simulink model "EPS_orbit_v5a"  (R2023b)
settings: Solver=FixedStepAuto  StartTime=0.0  StopTime=tsimulation  FixedStep=delta_t  RelTol=1e-3
undefined symbols (not defined in the file or in its folder): att, date, GS, juliandate, MODE, SP
libraries: dspmathops x17, vrlib x13, aerolibutil x11, sharedtransform x8, sharedutil x4, simulink_extras x1
(part 1 of 2)
settings Model: Creator=Ricardo  LastModifiedBy=lricc
settings SolverCC: AlgebraicLoopSolver=TrustRegion
settings OptimizationCC: ReuseModelBlockBuffer=off
settings DebuggingCC: UnconnectedInputMsg=warning  UnconnectedOutputMsg=warning  UnconnectedLineMsg=warning
settings ModelReferenceCC: EnableRefExpFcnMdlSchedulingChecks=on
settings RTWCC: DLArmComputeVersion=19.05

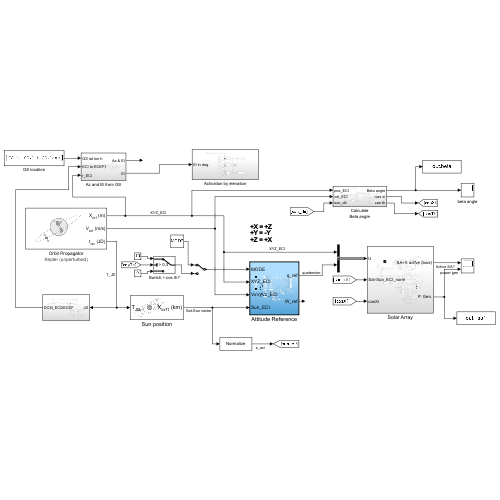
[thumbnail: Simulink's stored preview of the top-level diagram]
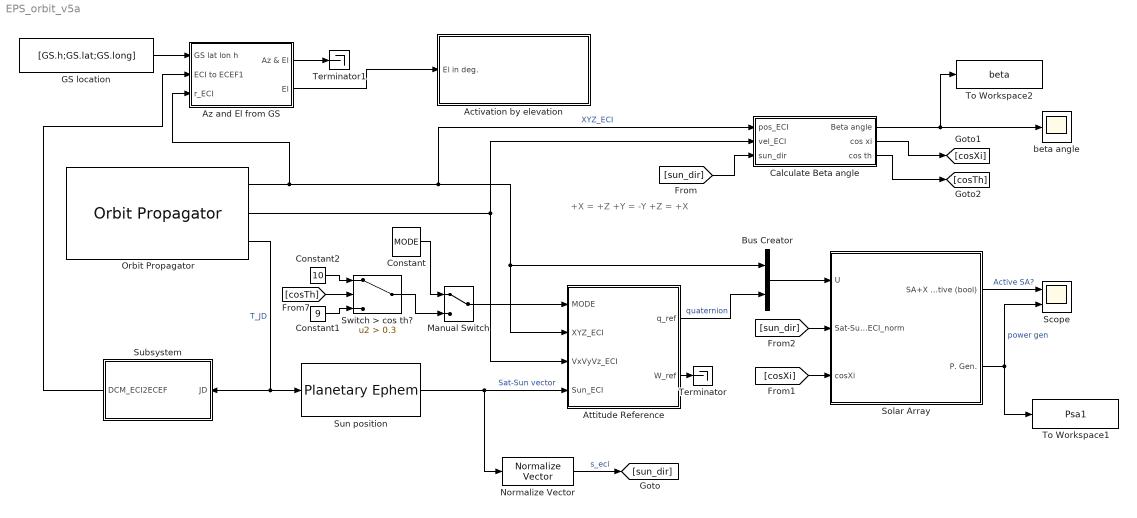
== system EPS_orbit_v5a ==
  note: +X = +Z
      | +Y = -Y
      | +Z = +X
  Activation by elevation : Subsystem
  Attitude Reference : Subsystem  TreatAsAtomicUnit=on
  Az and El from GS : Subsystem
  Bus Creator : BusCreator  Inputs=2
  Calculate Beta angle : Subsystem
  Constant : Constant  Value=MODE  OutDataTypeStr=int8
  Constant1 : Constant  Value=9
  Constant2 : Constant  Value=10
  GS location : Constant  Value=[GS.h;GS.lat;GS.long]
  Manual Switch : ManualSwitch
  Normalize Vector : vrlib/Utilities/Normalize Vector  maxzero=0
  Orbit Propagator : OrbitPropagator  startDate=juliandate(date.year, date.month, date.day, date.hour, date.minutes, date.seconds)  semiMajorAxis=orbit.a  eccentricity=orbit.e  inclination=orbit.i  raan=orbit.O  argPeriapsis=orbit.o  trueAnomaly=orbit.nu  inertialPosition=[3649700.0 3308200.0 -4676600.0]  inertialVelocity=[-2750.8 6666.4 2573.4]  fixedPosition=[-4142689.0 -2676864.7 -4669861.6]  fixedVelocity=[1452.7 -6720.7 2568.1]  customR=3396200  customMu=4.305e13  customJ2=1.0826269e-03  customOmega=4.06125949e-3
      settings: AttributesFormatString=%<propagator>
  Scope : Scope  NumInputPorts=2
  Solar Array : Subsystem
  Subsystem : Subsystem
  Sun position : PlanetaryEphem  target=Sun  outputVelocity=off
  Switch > cos th? : Switch  Criteria=u2 > Threshold  Threshold=0.3  SaturateOnIntegerOverflow=off  InputSameDT=off
  Terminator : Terminator
  Terminator1 : Terminator
  To Workspace1 : ToWorkspace  VariableName=Psa1  SaveFormat=Timeseries  SampleTime=-1
  To Workspace2 : ToWorkspace  VariableName=beta  SaveFormat=Timeseries  SampleTime=-1
  beta angle : Scope
  wires:
  Orbit Propagator/2 -> Attitude Reference/3(VxVyVz_ECI), Calculate Beta angle/2(vel_ECI)
  Orbit Propagator/1 -> Az and El from GS/3(r_ECI), Attitude Reference/2(XYZ_ECI), Bus Creator/1, Calculate Beta angle/1(pos_ECI)  "XYZ_ECI"
  Normalize Vector/1 -> [sun_dir]  "s_eci"
  Bus Creator/1 -> Solar Array/1(U)
  Sun position/1 -> Attitude Reference/4(Sun_ECI), Normalize Vector/1  "Sat-Sun vector"
  Solar Array/1(SA+X active (bool)) -> Scope/1  "Active SA?"
  Attitude Reference/1(q_ref) -> Bus Creator/2  "quaternion"
  Solar Array/2(P. Gen.) -> Scope/2, To Workspace1/1  "power gen"
  Orbit Propagator/3 -> Subsystem/1(JD), Sun position/1  "T_JD"
  Attitude Reference/2(W_ref) -> Terminator/1
  Constant/1 -> Manual Switch/1
  Calculate Beta angle/1(Beta angle) -> beta angle/1, To Workspace2/1
  [sun_dir] -> Calculate Beta angle/3(sun_dir)
  Calculate Beta angle/2(cos xi) -> [cosXi]
  [cosXi] -> Solar Array/3(cosXi)
  [sun_dir] -> Solar Array/2(Sat-Sun_ECI_norm)
  Manual Switch/1 -> Attitude Reference/1(MODE)
  Constant2/1 -> Switch > cos th?/1
  Constant1/1 -> Switch > cos th?/3
  [cosTh] -> Switch > cos th?/2
  Switch > cos th?/1 -> Manual Switch/2
  Calculate Beta angle/3(cos th) -> [cosTh]
  GS location/1 -> Az and El from GS/1(GS lat lon h)
  Subsystem/1(DCM_ECI2ECEF) -> Az and El from GS/2(ECI to ECEF1)
  Az and El from GS/1(Az & El) -> Terminator1/1
  Az and El from GS/2(El) -> Activation by elevation/1(El in deg.)

== system EPS_orbit_v5a/Activation by elevation ==
  El in deg. : Inport
  Constant1 : Constant
  Constant2 : Constant  Value=0
  Constant3 : Constant
  Constant4 : Constant  Value=0
  Constant5 : Constant
  Constant6 : Constant  Value=0
  Scope3 : Scope  NumInputPorts=3
  To Workspace1 : ToWorkspace  VariableName=el25  SaveFormat=Timeseries  SampleTime=-1
  To Workspace2 : ToWorkspace  VariableName=el00  SaveFormat=Timeseries  SampleTime=-1
  elevation>0 : Switch  Criteria=u2 > Threshold  SaturateOnIntegerOverflow=off  InputSameDT=off
  elevation>10 : Switch  Criteria=u2 > Threshold  Threshold=10  SaturateOnIntegerOverflow=off  InputSameDT=off
  elevation>25 : Switch  Criteria=u2 > Threshold  Threshold=25  SaturateOnIntegerOverflow=off  InputSameDT=off
  wires:
  Constant3/1 -> elevation>0/1
  Constant4/1 -> elevation>0/3
  elevation>0/1 -> To Workspace2/1, Scope3/1
  Constant2/1 -> elevation>10/3
  Constant1/1 -> elevation>10/1
  El in deg./1 -> elevation>25/2, elevation>10/2, elevation>0/2
  Constant6/1 -> elevation>25/3
  Constant5/1 -> elevation>25/1
  elevation>10/1 -> Scope3/2
  elevation>25/1 -> To Workspace1/1, Scope3/3

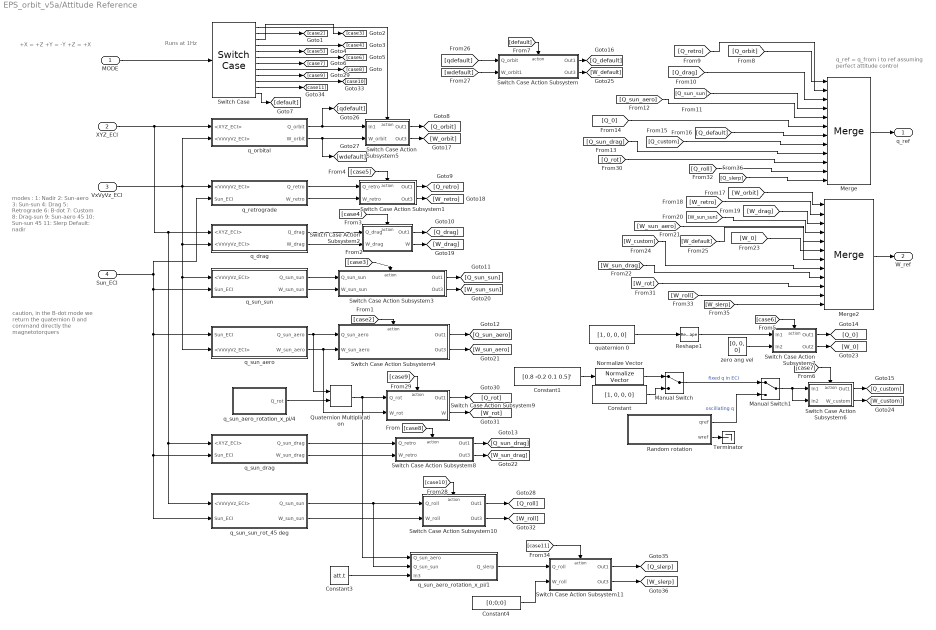
== system EPS_orbit_v5a/Attitude Reference ==
  note: caution, in the B-dot mode we return the quaternion 0 and command directly the magnetotorquers
  note: modes :
      | 1: Nadir
      | 2: Sun-aero
      | 3: Sun-sun
      | 4: Drag
      | 5: Retrograde
      | 6: B-dot
      | 7: Custom
      | 8: Drag-sun
      | 9: Sun-aero 45
      | 10: Sun-sun 45
      | 11: Slerp
      | Default: nadir
  note: q_ref  = q_from i to ref
      | assuming perfect attitude control
  note: Runs at 1Hz
  note: +X = +Z
      | +Y = -Y
      | +Z = +X
  MODE : Inport  OutMin=1  OutMax=100  OutDataTypeStr=int8
  XYZ_ECI : Inport  Port=2
  VxVyVz_ECI : Inport  Port=3
  Sun_ECI : Inport  Port=4
  Constant : Constant  Value=[1, 0, 0, 0]
  Constant1 : Constant  Value=[0.8 -0.2 0.1 0.5]'
  Constant3 : Constant  Value=att.t
  Constant4 : Constant  Value=[0;0;0]
  Manual Switch : ManualSwitch
  Manual Switch1 : ManualSwitch
  Merge : Merge  Inputs=12
  Merge2 : Merge  Inputs=12
  Normalize Vector : vrlib/Utilities/Normalize Vector  maxzero=0
  Quaternion Multiplication : aerolibutil/Quaternion Multiplication
  Random rotation : Subsystem
  Reshape1 : Reshape  OutputDimensionality=Column vector (2-D)
  Switch Case : SwitchCase  CaseConditions={1, 2, 3, 4, 5, 6, 7, 8, 9, 10, 11}
  Switch Case Action Subsystem : Subsystem  TreatAsAtomicUnit=on
  Switch Case Action Subsystem1 : Subsystem  TreatAsAtomicUnit=on
  Switch Case Action Subsystem10 : Subsystem  TreatAsAtomicUnit=on
  Switch Case Action Subsystem11 : Subsystem  TreatAsAtomicUnit=on
  Switch Case Action Subsystem2 : Subsystem  TreatAsAtomicUnit=on
  Switch Case Action Subsystem3 : Subsystem  TreatAsAtomicUnit=on
  Switch Case Action Subsystem4 : Subsystem  TreatAsAtomicUnit=on
  Switch Case Action Subsystem5 : Subsystem  TreatAsAtomicUnit=on
  Switch Case Action Subsystem6 : Subsystem  TreatAsAtomicUnit=on
  Switch Case Action Subsystem7 : Subsystem  TreatAsAtomicUnit=on
  Switch Case Action Subsystem8 : Subsystem  TreatAsAtomicUnit=on
  Switch Case Action Subsystem9 : Subsystem  TreatAsAtomicUnit=on
  Terminator : Terminator
  q_drag : Subsystem
  q_orbital : Subsystem
  q_retrograde : Subsystem
  q_sun_aero : Subsystem
  q_sun_aero_rotation_x_pi/1 : Subsystem
  q_sun_aero_rotation_x_pi/4 : Subsystem
  q_sun_drag : Subsystem
  q_sun_sun : Subsystem
  q_sun_sun_rot_45 deg : Subsystem
  quaternion 0 : Constant  Value=[1, 0, 0, 0]
  zero ang vel : Constant  Value=[0, 0, 0]
  q_ref : Outport  VectorParamsAs1DForOutWhenUnconnected=off
  W_ref : Outport  Port=2
  wires:
  quaternion 0/1 -> Reshape1/1
  Reshape1/1 -> Switch Case Action Subsystem7/1(In1)
  Constant/1 -> Manual Switch/2
  Constant1/1 -> Normalize Vector/1
  Normalize Vector/1 -> Manual Switch/1
  zero ang vel/1 -> Switch Case Action Subsystem7/2(In2)
  Manual Switch/1 -> Manual Switch1/1  "fixed q in ECI"
  Random rotation/1(qref) -> Manual Switch1/2  "oscillating q"
  Manual Switch1/1 -> Switch Case Action Subsystem6/2(In2), Switch Case Action Subsystem6/1(In1)
  [default] -> Switch Case Action Subsystem/Action
  Switch Case/7 -> [case7]
  Switch Case/4 -> [case4]
  Switch Case/5 -> [case5]
  [case3] -> Switch Case Action Subsystem3/Action
  [case5] -> Switch Case Action Subsystem1/Action
  Switch Case/3 -> [case3]
  Switch Case/2 -> [case2]
  q_drag/2(W_drag) -> Switch Case Action Subsystem2/2(W_drag)
  q_sun_drag/2(W_sun_drag) -> Switch Case Action Subsystem8/2(W_retro)
  q_sun_aero/2(W_sun_aero) -> Switch Case Action Subsystem9/2(W_rot), Switch Case Action Subsystem4/2(W_sun_aero)
  Switch Case/1 -> Switch Case Action Subsystem5/Action
  [case8] -> Switch Case Action Subsystem8/Action
  Switch Case/8 -> [case8]
  q_drag/1(Q_drag) -> Switch Case Action Subsystem2/1(Q_drag)
  Switch Case/12 -> [default]
  q_sun_sun/2(W_sun_sun) -> Switch Case Action Subsystem3/2(W_sun_sun)
  q_retrograde/2(W_retro) -> Switch Case Action Subsystem1/2(W_retro)
  q_sun_sun/1(Q_sun_sun) -> Switch Case Action Subsystem3/1(Q_sun_sun)
  q_sun_aero/1(Q_sun_aero) -> Quaternion Multiplication/1, Switch Case Action Subsystem4/1(Q_sun_aero)
  q_sun_drag/1(Q_sun_drag) -> Switch Case Action Subsystem8/1(Q_retro)
  Merge2/1 -> W_ref/1
  [case2] -> Switch Case Action Subsystem4/Action
  [case4] -> Switch Case Action Subsystem2/Action
  q_orbital/1(Q_orbit) -> [qdefault], Switch Case Action Subsystem5/1(In1)
  q_retrograde/1(Q_retro) -> Switch Case Action Subsystem1/1(Q_retro)
  q_orbital/2(W_orbit) -> [wdefault], Switch Case Action Subsystem5/2(W_orbit)
  Switch Case/6 -> [case6]
  VxVyVz_ECI/1 -> q_orbital/2(<VxVyVz_ECI>), q_retrograde/1(<VxVyVz_ECI>), q_drag/2(<VxVyVz_ECI>), q_sun_aero/2(<VxVyVz_ECI>), q_sun_sun/1(<VxVyVz_ECI>)
  Merge/1 -> q_ref/1
  MODE/1 -> Switch Case/1
  Random rotation/2(wref) -> Terminator/1
  [case6] -> Switch Case Action Subsystem7/Action
  [case7] -> Switch Case Action Subsystem6/Action
  Switch Case Action Subsystem5/1(Out1) -> [Q_orbit]
  [Q_orbit] -> Merge/1
  Switch Case Action Subsystem1/1(Out1) -> [Q_retro]
  [Q_retro] -> Merge/2
  Switch Case Action Subsystem2/1(Out1) -> [Q_drag]
  [Q_drag] -> Merge/3
  Switch Case Action Subsystem3/1(Out1) -> [Q_sun_sun]
  [Q_sun_sun] -> Merge/4
  Switch Case Action Subsystem4/1(Out1) -> [Q_sun_aero]
  [Q_sun_aero] -> Merge/5
  Switch Case Action Subsystem8/1(Out1) -> [Q_sun_drag]
  [Q_sun_drag] -> Merge/9
  Switch Case Action Subsystem7/1(Out1) -> [Q_0]
  [Q_0] -> Merge/6
  Switch Case Action Subsystem6/1(Out1) -> [Q_custom]
  [Q_custom] -> Merge/8
  Switch Case Action Subsystem/1(Out1) -> [Q_default]
  [Q_default] -> Merge/7
  Switch Case Action Subsystem5/2(Out3) -> [W_orbit]
  [W_orbit] -> Merge2/1
  Switch Case Action Subsystem1/2(Out3) -> [W_retro]
  [W_retro] -> Merge2/2
  Switch Case Action Subsystem2/2(W) -> [W_drag]
  [W_drag] -> Merge2/3
  Switch Case Action Subsystem3/2(Out3) -> [W_sun_sun]
  [W_sun_sun] -> Merge2/4
  Switch Case Action Subsystem4/2(Out3) -> [W_sun_aero]
  [W_sun_aero] -> Merge2/5
  Switch Case Action Subsystem8/2(Out3) -> [W_sun_drag]
  [W_sun_drag] -> Merge2/9
  Switch Case Action Subsystem7/2(Out2) -> [W_0]
  [W_0] -> Merge2/6
  Switch Case Action Subsystem6/2(W_custom) -> [W_custom]
  [W_custom] -> Merge2/8
  Switch Case Action Subsystem/2(Out3) -> [W_default]
  [W_default] -> Merge2/7
  [qdefault] -> Switch Case Action Subsystem/1(Q_orbit)
  [wdefault] -> Switch Case Action Subsystem/2(W_orbit1)
  q_sun_aero_rotation_x_pi/4/1(Q_rot) -> Quaternion Multiplication/2
  Quaternion Multiplication/1 -> q_sun_aero_rotation_x_pi/1/1(Q_sun_aero), Switch Case Action Subsystem9/1(Q_rot)
  Switch Case/9 -> [case9]
  [case9] -> Switch Case Action Subsystem9/Action
  Switch Case Action Subsystem9/1(Out1) -> [Q_rot]
  Switch Case Action Subsystem9/2(W) -> [W_rot]
  [Q_rot] -> Merge/10
  [W_rot] -> Merge2/10
  Sun_ECI/1 -> q_retrograde/2(Sun_ECI), q_sun_sun_rot_45 deg/2(Sun_ECI), q_sun_drag/2(Sun_ECI), q_sun_aero/1(Sun_ECI), q_sun_sun/2(Sun_ECI)
  q_sun_sun_rot_45 deg/1(Q_sun_sun) -> q_sun_aero_rotation_x_pi/1/2(Q_sun_sun), Switch Case Action Subsystem10/1(Q_roll)
  XYZ_ECI/1 -> q_sun_drag/1(<XYZ_ECI>), q_sun_sun_rot_45 deg/1(<VxVyVz_ECI>), q_drag/1(<XYZ_ECI>), q_orbital/1(<XYZ_ECI>)
  Switch Case Action Subsystem10/1(Out1) -> [Q_roll]
  [case10] -> Switch Case Action Subsystem10/Action
  q_sun_sun_rot_45 deg/2(W_sun_sun) -> Switch Case Action Subsystem10/2(W_roll)
  Switch Case Action Subsystem10/2(Out3) -> [W_roll]
  Switch Case/10 -> [case10]
  [Q_roll] -> Merge/11
  [W_roll] -> Merge2/11
  Switch Case/11 -> [case11]
  [W_slerp] -> Merge2/12
  Constant3/1 -> q_sun_aero_rotation_x_pi/1/3(In3)
  Switch Case Action Subsystem11/2(Out3) -> [W_slerp]
  [case11] -> Switch Case Action Subsystem11/Action
  Switch Case Action Subsystem11/1(Out1) -> [Q_slerp]
  q_sun_aero_rotation_x_pi/1/1(Q_slerp) -> Switch Case Action Subsystem11/1(Q_roll)
  Constant4/1 -> Switch Case Action Subsystem11/2(W_roll)
  [Q_slerp] -> Merge/12

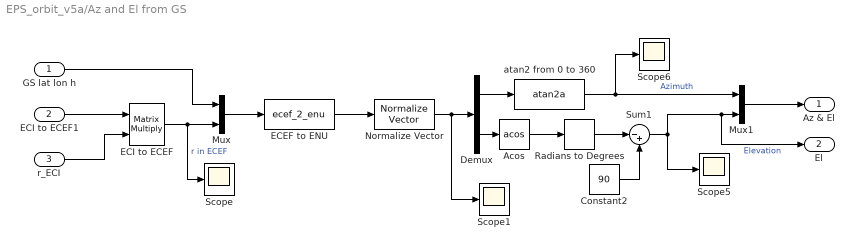
== system EPS_orbit_v5a/Az and El from GS ==
  GS lat lon h : Inport
  ECI to ECEF1 : Inport  Port=2
  r_ECI : Inport  Port=3
  Acos : Trigonometry  Operator=acos
  Constant2 : Constant  Value=90
  Demux : Demux  Outputs=[2,1]
  ECEF to ENU : MATLABFcn  MATLABFcn=ecef_2_enu  OutputDimensions=[3;1]  Output1D=off
  ECI to ECEF : Product  Multiplication=Matrix(*)
  Mux : Mux  Inputs=2
  Mux1 : Mux  Inputs=2
  Normalize Vector : vrlib/Utilities/Normalize Vector  maxzero=0
  Radians to Degrees : simulink_extras/Transformations/Radians to Degrees
  Scope{,1,5..6} (4 alike) : Scope
  Sum1 : Sum  Inputs=|-+
  atan2 from 0 to 360 : MATLABFcn  MATLABFcn=atan2a
  Az & El : Outport
  El : Outport  Port=2
  wires:
  atan2 from 0 to 360/1 -> Scope6/1, Mux1/1  "Azimuth"
  ECEF to ENU/1 -> Normalize Vector/1
  GS lat lon h/1 -> Mux/1
  Acos/1 -> Radians to Degrees/1
  ECI to ECEF1/1 -> ECI to ECEF/1
  ECI to ECEF/1 -> Scope/1, Mux/2  "r in ECEF"
  Demux/2 -> Acos/1
  Mux/1 -> ECEF to ENU/1
  Sum1/1 -> Scope5/1, El/1, Mux1/2  "Elevation"
  Normalize Vector/1 -> Scope1/1, Demux/1
  Demux/1 -> atan2 from 0 to 360/1
  Radians to Degrees/1 -> Sum1/1
  Constant2/1 -> Sum1/2
  r_ECI/1 -> ECI to ECEF/2
  Mux1/1 -> Az & El/1

== system EPS_orbit_v5a/Calculate Beta angle ==
  note: xi is calculated for the Albedo
  pos_ECI : Inport
  vel_ECI : Inport  Port=2
  sun_dir : Inport  Port=3
  Acos : Trigonometry  Operator=acos
  Constant1 : Constant  Value=90
  Cross Product : vrlib/Utilities/Cross Product
  Dot Product : DotProduct  OutDataTypeStr=Inherit: Inherit via internal rule
  Dot Product1 : DotProduct  OutDataTypeStr=Inherit: Inherit via internal rule
  Gain : Gain  Gain=180/pi
  Normalize Vector1 : vrlib/Utilities/Normalize Vector  maxzero=0
  Normalize Vector2 : vrlib/Utilities/Normalize Vector  maxzero=0
  Product : Product
  Scope : Scope  NumInputPorts=2
  Sin : Trigonometry
  Sum : Sum  Inputs=|-+
  Beta angle : Outport
  cos xi : Outport  Port=2
  cos th : Outport  Port=3
  wires:
  vel_ECI/1 -> Cross Product/2
  Dot Product/1 -> Acos/1
  Acos/1 -> Sin/1, Gain/1
  Normalize Vector1/1 -> Dot Product/2  "x"
  Gain/1 -> Sum/1
  sun_dir/1 -> Dot Product1/2, Dot Product/1
  Cross Product/1 -> Normalize Vector1/1
  Constant1/1 -> Sum/2
  pos_ECI/1 -> Normalize Vector2/1, Cross Product/1
  Sum/1 -> Beta angle/1
  Dot Product1/1 -> cos th/1, Product/2, Scope/2  "cos(theta)"
  Normalize Vector2/1 -> Dot Product1/1  "x"
  Sin/1 -> Product/1  "cos(beta)"
  Product/1 -> Scope/1, cos xi/1

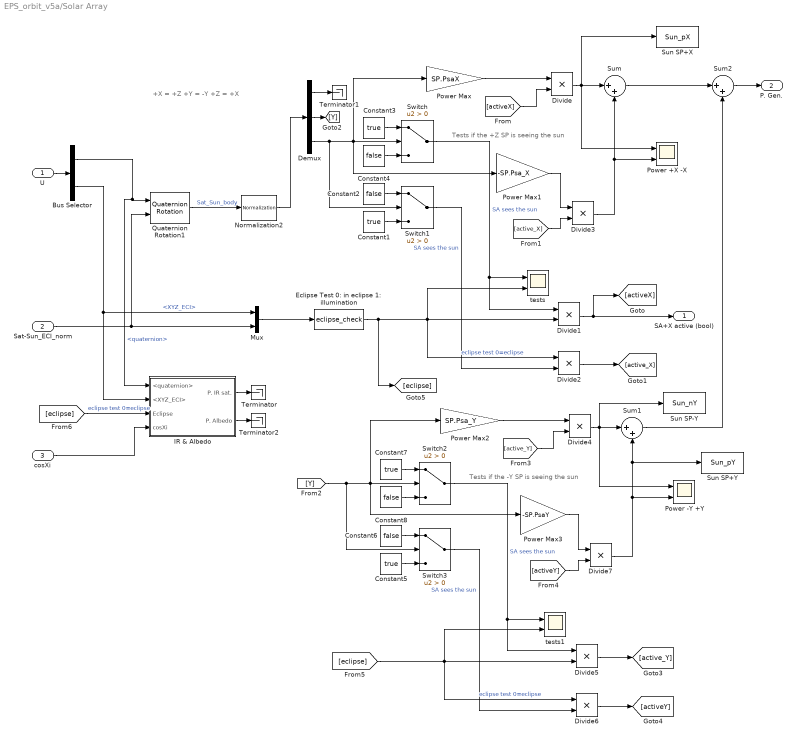
== system EPS_orbit_v5a/Solar Array ==
  note: Tests if the +Z SP is seeing the sun
  note: +X = +Z
      | +Y = -Y
      | +Z = +X
  note: Tests if the -Y SP is seeing the sun
  U : Inport
  Sat-Sun_ECI_norm : Inport  Port=2
  cosXi : Inport  Port=3
  Bus Selector : BusSelector  OutputSignals=quaternion,XYZ_ECI
  Constant{1,3,5,7} (4 alike) : Constant  Value=true
  Constant{2,4,6,8} (4 alike) : Constant  Value=false
  Demux : Demux  Outputs=3
  Divide{,1..7} (8 alike) : Product  Inputs=**
  Eclipse Test 0: in eclipse 1: illumination : MATLABFcn  MATLABFcn=eclipse_check
  IR & Albedo : Subsystem
  Mux : Mux  Inputs=2
  Normalization2 : dspmathops/Normalization  NormType=2-norm  Bias=1e-10  NormOver=Each column  Dimension=1  roundingMode=Floor  overflowMode=off  accumDataTypeStr=Inherit: Same as product output  accumLastDataTypeStr=Inherit: Same as product output  outputDataTypeStr=Inherit: Same as product output  outputMin=[]  outputMax=[]  outputLastDataTypeStr=Inherit: Same as product output
  Power +X -X : Scope  NumInputPorts=2
  Power -Y +Y : Scope  NumInputPorts=2
  Power Max : Gain  Gain=SP.PsaX
  Power Max1 : Gain  Gain=-SP.Psa_X
  Power Max2 : Gain  Gain=SP.Psa_Y
  Power Max3 : Gain  Gain=-SP.PsaY
  Quaternion Rotation1 : aerolibutil/Quaternion Rotation
  Sum : Sum  Inputs=|++
  Sum1 : Sum  Inputs=|++
  Sum2 : Sum  Inputs=|++
  Sun SP+X : ToWorkspace  VariableName=Sun_pX  SaveFormat=Timeseries  SampleTime=1
      settings: Save2DSignal=2-D array (concatenate along first dimension)
  Sun SP+Y : ToWorkspace  VariableName=Sun_pY  SaveFormat=Timeseries  SampleTime=1
      settings: Save2DSignal=2-D array (concatenate along first dimension)
  Sun SP-Y : ToWorkspace  VariableName=Sun_nY  SaveFormat=Timeseries  SampleTime=1
      settings: Save2DSignal=2-D array (concatenate along first dimension)
  Switch{,1..3} (4 alike) : Switch  Criteria=u2 > Threshold  SaturateOnIntegerOverflow=off  InputSameDT=off
  Terminator : Terminator
  Terminator1 : Terminator
  Terminator2 : Terminator
  tests : Scope  NumInputPorts=2
  tests1 : Scope  NumInputPorts=2
  SA+X active (bool) : Outport  VectorParamsAs1DForOutWhenUnconnected=off
  P. Gen. : Outport  Port=2
  wires:
  Switch/1 -> Divide1/1, tests/1  "SA sees the sun"
  U/1 -> Bus Selector/1
  Bus Selector/1 -> Quaternion Rotation1/1, IR & Albedo/1(<quaternion>)  "<quaternion>"
  Quaternion Rotation1/1 -> Normalization2/1  "Sat_Sun_body"
  Constant3/1 -> Switch/1
  Demux/2 -> [Y]
  Demux/1 -> Terminator1/1
  Bus Selector/2 -> IR & Albedo/2(<XYZ_ECI>), Mux/1  "<XYZ_ECI>"
  Divide1/1 -> [activeX], SA+X active (bool)/1
  Constant4/1 -> Switch/3
  Normalization2/1 -> Demux/1
  Divide/1 -> Sun SP+X/1, Power +X -X/1, Sum/1
  Power Max/1 -> Divide/1
  [activeX] -> Divide/2
  Sat-Sun_ECI_norm/1 -> Quaternion Rotation1/2, Mux/2
  Mux/1 -> Eclipse Test 0: in eclipse 1: illumination/1
  Eclipse Test 0: in eclipse 1: illumination/1 -> [eclipse], Divide2/1, tests/2, Divide1/2  "eclipse test 0=eclipse"
  Demux/3 -> Switch1/2, Power Max1/1, Power Max/1, Switch/2
  Constant2/1 -> Switch1/1
  Constant1/1 -> Switch1/3
  Switch1/1 -> Divide2/2  "SA sees the sun"
  Divide2/1 -> [active_X]
  [active_X] -> Divide3/2
  Power Max1/1 -> Divide3/1
  Divide3/1 -> Sum/2, Power +X -X/2
  Sum/1 -> Sum2/1
  [Y] -> Switch3/2, Power Max3/1, Power Max2/1, Switch2/2
  [eclipse] -> Divide6/1, tests1/2, Divide5/2  "eclipse test 0=eclipse"
  [active_Y] -> Divide4/2
  Constant7/1 -> Switch2/1
  Divide5/1 -> [active_Y]
  Constant8/1 -> Switch2/3
  Switch2/1 -> Divide5/1, tests1/1  "SA sees the sun"
  Sum1/1 -> Sum2/2
  Divide6/1 -> [activeY]
  Divide4/1 -> Sun SP-Y/1, Power -Y +Y/1, Sum1/1
  Switch3/1 -> Divide6/2  "SA sees the sun"
  Constant6/1 -> Switch3/1
  Power Max2/1 -> Divide4/1
  [activeY] -> Divide7/2
  Power Max3/1 -> Divide7/1
  Divide7/1 -> Power -Y +Y/2, Sun SP+Y/1, Sum1/2
  Constant5/1 -> Switch3/3
  Sum2/1 -> P. Gen./1
  [eclipse] -> IR & Albedo/3(Eclipse)  "eclipse test 0=eclipse"
  cosXi/1 -> IR & Albedo/4(cosXi)
  IR & Albedo/1(P. IR sat.) -> Terminator/1
  IR & Albedo/2(P. Albedo) -> Terminator2/1

== system EPS_orbit_v5a/Subsystem ==
  JD : Inport
  ECI_2_ECEF : MATLABFcn  MATLABFcn=eci2ecef  OutputDimensions=[3,3]  Output1D=off
  JD to UTC : MATLAB Function  TreatAsAtomicUnit=on
  Reshape : Reshape
  Scope : Scope
  Scope1 : Scope
  Signal logging : ToWorkspace  VariableName=T_UTC  SaveFormat=Timeseries  SampleTime=1
      settings: Save2DSignal=2-D array (concatenate along first dimension)
  Signal logging1 : ToWorkspace  VariableName=T_JD  SaveFormat=Timeseries  SampleTime=1
      settings: Save2DSignal=2-D array (concatenate along first dimension)
  DCM_ECI2ECEF : Outport
  wires:
  JD/1 -> Signal logging1/1, JD to UTC/1(JD)
  Reshape/1 -> Scope/1, ECI_2_ECEF/1, Signal logging/1
  JD to UTC/1(Time_UTC) -> Reshape/1
  ECI_2_ECEF/1 -> Scope1/1, DCM_ECI2ECEF/1

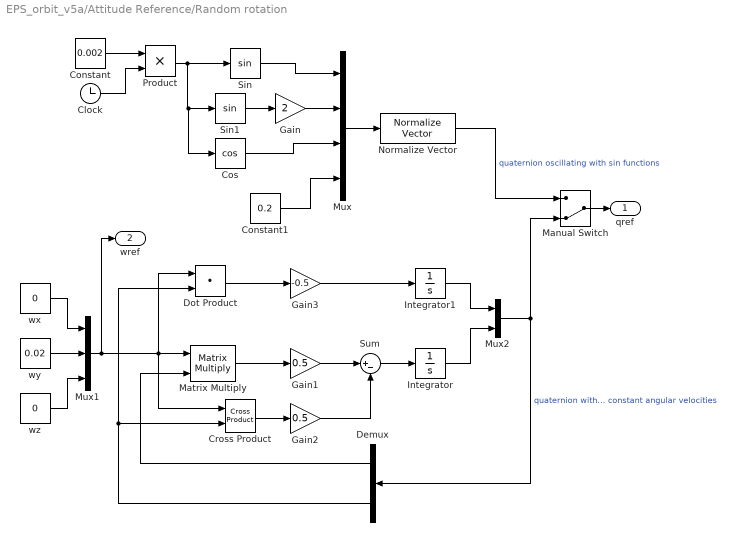
== system EPS_orbit_v5a/Attitude Reference/Random rotation ==
  Clock : Clock
      settings: Decimation=TimeStep
  Constant : Constant  Value=0.002
  Constant1 : Constant  Value=0.2
  Cos : Trigonometry  Operator=cos
  Cross Product : vrlib/Utilities/Cross Product
  Demux : Demux  Outputs=[1;3]
  Dot Product : DotProduct  OutDataTypeStr=Inherit: Inherit via internal rule
  Gain : Gain  Gain=2
  Gain1 : Gain  Gain=0.5
  Gain2 : Gain  Gain=0.5
  Gain3 : Gain  Gain=-0.5
  Integrator : Integrator  InitialCondition=[0;0;0]
  Integrator1 : Integrator  InitialCondition=1
  Manual Switch : ManualSwitch  CurrentSetting=0
  Matrix Multiply : Product  Multiplication=Matrix(*)
  Mux : Mux
  Mux1 : Mux  Inputs=3
  Mux2 : Mux  Inputs=[1;3]
  Normalize Vector : vrlib/Utilities/Normalize Vector  maxzero=0
  Product : Product
  Sin : Trigonometry
  Sin1 : Trigonometry
  Sum : Sum  Inputs=|+-
  wx : Constant  Value=0
  wy : Constant  Value=0.02
  wz : Constant  Value=0
  qref : Outport
  wref : Outport  Port=2
  wires:
  Mux/1 -> Normalize Vector/1
  Normalize Vector/1 -> Manual Switch/1  "quaternion oscillating with sin functions"
  Constant/1 -> Product/1
  Clock/1 -> Product/2
  Product/1 -> Cos/1, Sin1/1, Sin/1
  Sin/1 -> Mux/1
  Sin1/1 -> Gain/1
  Gain/1 -> Mux/2
  Cos/1 -> Mux/3
  Constant1/1 -> Mux/4
  Manual Switch/1 -> qref/1
  wx/1 -> Mux1/1
  wy/1 -> Mux1/2
  wz/1 -> Mux1/3
  Mux1/1 -> wref/1, Dot Product/1, Cross Product/1, Matrix Multiply/1
  Matrix Multiply/1 -> Gain1/1
  Gain1/1 -> Sum/1
  Sum/1 -> Integrator/1
  Integrator/1 -> Mux2/2
  Mux2/1 -> Demux/1, Manual Switch/2  "quaternion with constant angular velocities"
  Demux/1 -> Matrix Multiply/2
  Cross Product/1 -> Gain2/1
  Gain2/1 -> Sum/2
  Dot Product/1 -> Gain3/1
  Gain3/1 -> Integrator1/1
  Integrator1/1 -> Mux2/1
  Demux/2 -> Cross Product/2, Dot Product/2

== system EPS_orbit_v5a/Attitude Reference/Switch Case Action Subsystem ==
  Q_orbit : Inport
  W_orbit1 : Inport  Port=2
  Action Port : ActionPort  ActionPortLabel=default:
  Out1 : Outport  VectorParamsAs1DForOutWhenUnconnected=off
  Out3 : Outport  Port=2  VectorParamsAs1DForOutWhenUnconnected=off
  wires:
  Q_orbit/1 -> Out1/1
  W_orbit1/1 -> Out3/1

== system EPS_orbit_v5a/Attitude Reference/Switch Case Action Subsystem1 ==
  Q_retro : Inport
  W_retro : Inport  Port=2
  Action Port : ActionPort  ActionPortLabel=case [ 5 ]:
  Out1 : Outport  VectorParamsAs1DForOutWhenUnconnected=off
  Out3 : Outport  Port=2  VectorParamsAs1DForOutWhenUnconnected=off
  wires:
  Q_retro/1 -> Out1/1
  W_retro/1 -> Out3/1

== system EPS_orbit_v5a/Attitude Reference/Switch Case Action Subsystem10 ==
  note: from I to SS
  Q_roll : Inport
  W_roll : Inport  Port=2
  Action Port : ActionPort  ActionPortLabel=case [ 10 ]:
  Out1 : Outport  VectorParamsAs1DForOutWhenUnconnected=off
  Out3 : Outport  Port=2  VectorParamsAs1DForOutWhenUnconnected=off
  wires:
  Q_roll/1 -> Out1/1
  W_roll/1 -> Out3/1

== system EPS_orbit_v5a/Attitude Reference/Switch Case Action Subsystem11 ==
  note: from I to SS
  Q_roll : Inport
  W_roll : Inport  Port=2
  Action Port : ActionPort  ActionPortLabel=case [ 11 ]:
  Out1 : Outport  VectorParamsAs1DForOutWhenUnconnected=off
  Out3 : Outport  Port=2  VectorParamsAs1DForOutWhenUnconnected=off
  wires:
  Q_roll/1 -> Out1/1
  W_roll/1 -> Out3/1

== system EPS_orbit_v5a/Attitude Reference/Switch Case Action Subsystem2 ==
  note: q from I to O + rotation
  Q_drag : Inport
  W_drag : Inport  Port=2
  Action Port : ActionPort  ActionPortLabel=case [ 4 ]:
  Out1 : Outport  VectorParamsAs1DForOutWhenUnconnected=off
  W : Outport  Port=2
  wires:
  Q_drag/1 -> Out1/1
  W_drag/1 -> W/1

== system EPS_orbit_v5a/Attitude Reference/Switch Case Action Subsystem3 ==
  Q_sun_sun : Inport
  W_sun_sun : Inport  Port=2
  Action Port : ActionPort  ActionPortLabel=case [ 3 ]:
  Out1 : Outport  VectorParamsAs1DForOutWhenUnconnected=off
  Out3 : Outport  Port=2  VectorParamsAs1DForOutWhenUnconnected=off
  wires:
  Q_sun_sun/1 -> Out1/1
  W_sun_sun/1 -> Out3/1

== system EPS_orbit_v5a/Attitude Reference/Switch Case Action Subsystem4 ==
  Q_sun_aero : Inport
  W_sun_aero : Inport  Port=2
  Action Port : ActionPort  ActionPortLabel=case [ 2 ]:
  Out1 : Outport  VectorParamsAs1DForOutWhenUnconnected=off
  Out3 : Outport  Port=2  VectorParamsAs1DForOutWhenUnconnected=off
  wires:
  Q_sun_aero/1 -> Out1/1
  W_sun_aero/1 -> Out3/1

== system EPS_orbit_v5a/Attitude Reference/Switch Case Action Subsystem5 ==
  In1 : Inport
  W_orbit : Inport  Port=2
  Action Port : ActionPort  ActionPortLabel=case [ 1 ]:
  Out1 : Outport  VectorParamsAs1DForOutWhenUnconnected=off
  Out3 : Outport  Port=2  VectorParamsAs1DForOutWhenUnconnected=off
  wires:
  In1/1 -> Out1/1
  W_orbit/1 -> Out3/1

== system EPS_orbit_v5a/Attitude Reference/Switch Case Action Subsystem6 ==
  In1 : Inport
  In2 : Inport  Port=2
  Action Port : ActionPort  ActionPortLabel=case [ 7 ]:
  Derivative : Derivative
  Matrix Multiply : Product  Multiplication=Matrix(*)
  Quaternions to Direction Cosine Matrix : sharedtransform/Quaternions to  Direction Cosine Matrix  aMode=aMode
  Transpose : Math  Operator=transpose
  Transpose1 : Math  Operator=transpose
  gets vector from Skew Matrix : MATLABFcn  MATLABFcn=vec_from_skew
  Out1 : Outport  VectorParamsAs1DForOutWhenUnconnected=off
  W_custom : Outport  Port=2
  wires:
  In1/1 -> Out1/1
  In2/1 -> Quaternions to Direction Cosine Matrix/1
  Quaternions to Direction Cosine Matrix/1 -> Transpose1/1
  Matrix Multiply/1 -> gets vector from Skew Matrix/1
  Transpose/1 -> Derivative/1
  gets vector from Skew Matrix/1 -> W_custom/1
  Derivative/1 -> Matrix Multiply/1
  Transpose1/1 -> Transpose/1, Matrix Multiply/2

== system EPS_orbit_v5a/Attitude Reference/Switch Case Action Subsystem7 ==
  In1 : Inport
  In2 : Inport  Port=2
  Action Port : ActionPort  ActionPortLabel=case [ 6 ]:
  Out1 : Outport  VectorParamsAs1DForOutWhenUnconnected=off
  Out2 : Outport  Port=2  VectorParamsAs1DForOutWhenUnconnected=off
  wires:
  In1/1 -> Out1/1
  In2/1 -> Out2/1

== system EPS_orbit_v5a/Attitude Reference/Switch Case Action Subsystem8 ==
  Q_retro : Inport
  W_retro : Inport  Port=2
  Action Port : ActionPort  ActionPortLabel=case [ 8 ]:
  Out1 : Outport  VectorParamsAs1DForOutWhenUnconnected=off
  Out3 : Outport  Port=2  VectorParamsAs1DForOutWhenUnconnected=off
  wires:
  Q_retro/1 -> Out1/1
  W_retro/1 -> Out3/1

== system EPS_orbit_v5a/Attitude Reference/Switch Case Action Subsystem9 ==
  note: q from I to O + rotation
  Q_rot : Inport
  W_rot : Inport  Port=2
  Action Port : ActionPort  ActionPortLabel=case [ 9 ]:
  Out1 : Outport  VectorParamsAs1DForOutWhenUnconnected=off
  W : Outport  Port=2
  wires:
  Q_rot/1 -> Out1/1
  W_rot/1 -> W/1

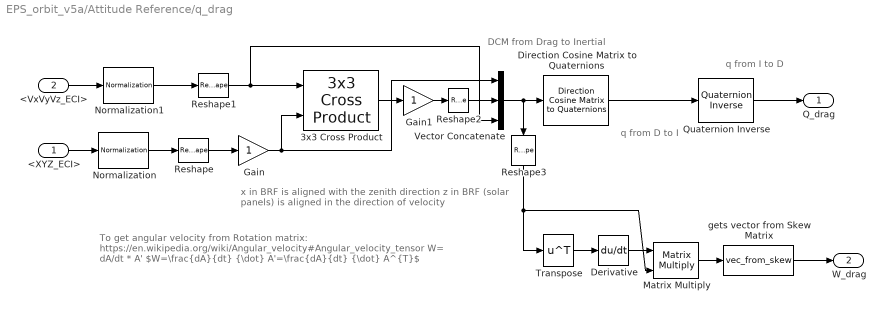
== system EPS_orbit_v5a/Attitude Reference/q_drag ==
  note: x in BRF is aligned with the zenith direction
      | z in BRF (solar panels) is aligned in the direction of velocity
  note: DCM from Drag to Inertial
  note: q from D to I
  note: q from I to D
  note: To get angular velocity from Rotation matrix:
      | https://en.wikipedia.org/wiki/Angular_velocity#Angular_velocity_tensor
      | W= dA/dt * A'
      | $W=\frac{dA}{dt} {\dot} A'=\frac{dA}{dt} {\dot} A^{T}$
  <XYZ_ECI> : Inport
  <VxVyVz_ECI> : Inport  Port=2
  3x3 Cross Product : sharedutil/3x3 Cross Product  aMode=aMode
  Derivative : Derivative
  Direction Cosine Matrix to Quaternions : sharedtransform/Direction Cosine Matrix  to Quaternions  aMode=0  action=None  tolerance=eps(2)
  Gain : Gain
  Gain1 : Gain
  Matrix Multiply : Product  Multiplication=Matrix(*)
  Normalization : dspmathops/Normalization  NormType=2-norm  Bias=1e-10  NormOver=Each column  Dimension=1  roundingMode=Floor  overflowMode=off  accumDataTypeStr=Inherit: Same as product output  accumLastDataTypeStr=Inherit: Same as product output  outputDataTypeStr=Inherit: Same as product output  outputMin=[]  outputMax=[]  outputLastDataTypeStr=Inherit: Same as product output
  Normalization1 : dspmathops/Normalization  NormType=2-norm  Bias=1e-10  NormOver=Each column  Dimension=1  roundingMode=Floor  overflowMode=off  accumDataTypeStr=Inherit: Same as product output  accumLastDataTypeStr=Inherit: Same as product output  outputDataTypeStr=Inherit: Same as product output  outputMin=[]  outputMax=[]  outputLastDataTypeStr=Inherit: Same as product output
  Quaternion Inverse : aerolibutil/Quaternion Inverse
  Reshape : Reshape  OutputDimensionality=Column vector (2-D)
  Reshape1 : Reshape  OutputDimensionality=Column vector (2-D)
  Reshape2 : Reshape  OutputDimensionality=Column vector (2-D)
  Reshape3 : Reshape  OutputDimensionality=Customize  OutputDimensions=[3,3]
  Transpose : Math  Operator=transpose
  Vector Concatenate : Concatenate  NumInputs=3  Mode=Multidimensional array  ConcatenateDimension=2
  gets vector from Skew Matrix : MATLABFcn  MATLABFcn=vec_from_skew
  Q_drag : Outport  VectorParamsAs1DForOutWhenUnconnected=off
  W_drag : Outport  Port=2
  wires:
  Normalization/1 -> Reshape/1
  Normalization1/1 -> Reshape1/1
  <VxVyVz_ECI>/1 -> Normalization1/1
  Reshape1/1 -> Vector Concatenate/3, 3x3 Cross Product/1
  <XYZ_ECI>/1 -> Normalization/1
  Reshape/1 -> Gain/1
  Gain/1 -> Vector Concatenate/1, 3x3 Cross Product/2
  Direction Cosine Matrix to Quaternions/1 -> Quaternion Inverse/1
  3x3 Cross Product/1 -> Gain1/1
  Gain1/1 -> Reshape2/1
  Quaternion Inverse/1 -> Q_drag/1
  Vector Concatenate/1 -> Reshape3/1, Direction Cosine Matrix to Quaternions/1
  gets vector from Skew Matrix/1 -> W_drag/1
  Matrix Multiply/1 -> gets vector from Skew Matrix/1
  Transpose/1 -> Derivative/1
  Derivative/1 -> Matrix Multiply/1
  Reshape2/1 -> Vector Concatenate/2
  Reshape3/1 -> Matrix Multiply/2, Transpose/1

== system EPS_orbit_v5a/Attitude Reference/q_orbital ==
  note: DCM from Orbital to Inertial
  note: q from O to I
  note: q from I to O
  note: To get angular velocity from Rotation matrix:
      | https://en.wikipedia.org/wiki/Angular_velocity#Angular_velocity_tensor
      | W= dA/dt * A'
      | $W=\frac{dA}{dt} {\dot} A'=\frac{dA}{dt} {\dot} A^{T}$
  <XYZ_ECI> : Inport
  <VxVyVz_ECI> : Inport  Port=2
  3x3 Cross Product : sharedutil/3x3 Cross Product  aMode=aMode
  Derivative : Derivative
  Direction Cosine Matrix to Quaternions : sharedtransform/Direction Cosine Matrix  to Quaternions  aMode=0  action=None  tolerance=eps(2)
  Gain : Gain
  Gain1 : Gain  Gain=-1
  Matrix Multiply : Product  Multiplication=Matrix(*)
  Normalization : dspmathops/Normalization  NormType=2-norm  Bias=1e-10  NormOver=Each column  Dimension=1  roundingMode=Floor  overflowMode=off  accumDataTypeStr=Inherit: Same as product output  accumLastDataTypeStr=Inherit: Same as product output  outputDataTypeStr=Inherit: Same as product output  outputMin=[]  outputMax=[]  outputLastDataTypeStr=Inherit: Same as product output
  Normalization1 : dspmathops/Normalization  NormType=2-norm  Bias=1e-10  NormOver=Each column  Dimension=1  roundingMode=Floor  overflowMode=off  accumDataTypeStr=Inherit: Same as product output  accumLastDataTypeStr=Inherit: Same as product output  outputDataTypeStr=Inherit: Same as product output  outputMin=[]  outputMax=[]  outputLastDataTypeStr=Inherit: Same as product output
  Quaternion Inverse : aerolibutil/Quaternion Inverse
  Reshape : Reshape  OutputDimensionality=Column vector (2-D)
  Reshape1 : Reshape  OutputDimensionality=Column vector (2-D)
  Reshape2 : Reshape  OutputDimensionality=Column vector (2-D)
  Reshape3 : Reshape  OutputDimensionality=Customize  OutputDimensions=[3,3]
  Transpose : Math  Operator=transpose
  Vector Concatenate : Concatenate  NumInputs=3  Mode=Multidimensional array  ConcatenateDimension=2
  gets vector from Skew Matrix : MATLABFcn  MATLABFcn=vec_from_skew
  Q_orbit : Outport  VectorParamsAs1DForOutWhenUnconnected=off
  W_orbit : Outport  Port=2
  wires:
  Normalization/1 -> Reshape/1
  Normalization1/1 -> Reshape1/1
  <VxVyVz_ECI>/1 -> Normalization1/1
  Reshape1/1 -> 3x3 Cross Product/1, Vector Concatenate/1
  <XYZ_ECI>/1 -> Normalization/1
  Reshape/1 -> Gain/1
  Gain/1 -> 3x3 Cross Product/2, Vector Concatenate/3
  Direction Cosine Matrix to Quaternions/1 -> Quaternion Inverse/1
  3x3 Cross Product/1 -> Gain1/1
  Gain1/1 -> Reshape2/1
  Quaternion Inverse/1 -> Q_orbit/1
  Vector Concatenate/1 -> Reshape3/1, Direction Cosine Matrix to Quaternions/1
  gets vector from Skew Matrix/1 -> W_orbit/1
  Matrix Multiply/1 -> gets vector from Skew Matrix/1
  Transpose/1 -> Derivative/1
  Derivative/1 -> Matrix Multiply/1
  Reshape2/1 -> Vector Concatenate/2
  Reshape3/1 -> Matrix Multiply/2, Transpose/1

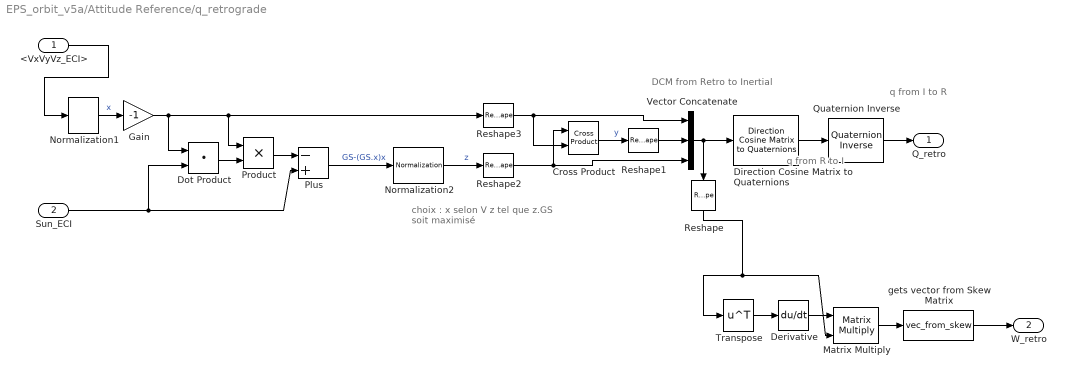
== system EPS_orbit_v5a/Attitude Reference/q_retrograde ==
  note: q from I to R
  note: q from R to I
  note: DCM from Retro to Inertial
  note: choix :
      | x selon V
      | z tel que z.GS soit maximisé
  <VxVyVz_ECI> : Inport
  Sun_ECI : Inport  Port=2
  Cross Product : vrlib/Utilities/Cross Product
  Derivative : Derivative
  Direction Cosine Matrix to Quaternions : sharedtransform/Direction Cosine Matrix  to Quaternions  aMode=0  action=None  tolerance=eps(2)
  Dot Product : DotProduct  OutDataTypeStr=Inherit: Inherit via internal rule
  Gain : Gain  Gain=-1
  Matrix Multiply : Product  Multiplication=Matrix(*)
  Normalization1 : dspmathops/Normalization  NormType=2-norm  Bias=1e-10  NormOver=Each column  Dimension=1  roundingMode=Floor  overflowMode=off  accumDataTypeStr=Inherit: Same as product output  accumLastDataTypeStr=Inherit: Same as product output  outputDataTypeStr=Inherit: Same as product output  outputMin=[]  outputMax=[]  outputLastDataTypeStr=Inherit: Same as product output
  Normalization2 : dspmathops/Normalization  NormType=2-norm  Bias=1e-10  NormOver=Each column  Dimension=1  roundingMode=Floor  overflowMode=off  accumDataTypeStr=Inherit: Same as product output  accumLastDataTypeStr=Inherit: Same as product output  outputDataTypeStr=Inherit: Same as product output  outputMin=[]  outputMax=[]  outputLastDataTypeStr=Inherit: Same as product output
  Plus : Sum  Inputs=-+
  Product : Product
  Quaternion Inverse : aerolibutil/Quaternion Inverse
  Reshape : Reshape  OutputDimensionality=Customize  OutputDimensions=[3,3]
  Reshape1 : Reshape  OutputDimensionality=Column vector (2-D)
  Reshape2 : Reshape  OutputDimensionality=Column vector (2-D)
  Reshape3 : Reshape  OutputDimensionality=Column vector (2-D)
  Transpose : Math  Operator=transpose
  Vector Concatenate : Concatenate  NumInputs=3  Mode=Multidimensional array  ConcatenateDimension=2
  gets vector from Skew Matrix : MATLABFcn  MATLABFcn=vec_from_skew
  Q_retro : Outport  VectorParamsAs1DForOutWhenUnconnected=off
  W_retro : Outport  Port=2
  wires:
  Quaternion Inverse/1 -> Q_retro/1
  Reshape2/1 -> Vector Concatenate/3, Cross Product/1
  Reshape3/1 -> Vector Concatenate/1, Cross Product/2
  Product/1 -> Plus/1
  Dot Product/1 -> Product/2
  Cross Product/1 -> Reshape1/1  "y"
  Normalization2/1 -> Reshape2/1  "z"
  Plus/1 -> Normalization2/1  "GS-(GS.x)x"
  Sun_ECI/1 -> Dot Product/2, Plus/2
  Direction Cosine Matrix to Quaternions/1 -> Quaternion Inverse/1
  Normalization1/1 -> Gain/1  "x"
  <VxVyVz_ECI>/1 -> Normalization1/1
  Reshape1/1 -> Vector Concatenate/2
  Gain/1 -> Dot Product/1, Product/1, Reshape3/1
  Vector Concatenate/1 -> Direction Cosine Matrix to Quaternions/1, Reshape/1
  gets vector from Skew Matrix/1 -> W_retro/1
  Matrix Multiply/1 -> gets vector from Skew Matrix/1
  Derivative/1 -> Matrix Multiply/1
  Transpose/1 -> Derivative/1
  Reshape/1 -> Transpose/1, Matrix Multiply/2

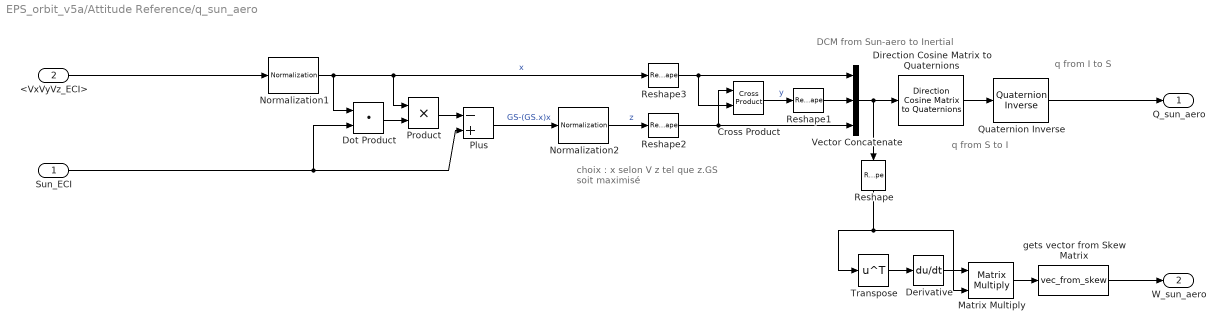
== system EPS_orbit_v5a/Attitude Reference/q_sun_aero ==
  note: q from I to S
  note: q from S to I
  note: DCM from Sun-aero to Inertial
  note: choix :
      | x selon V
      | z tel que z.GS soit maximisé
  Sun_ECI : Inport
  <VxVyVz_ECI> : Inport  Port=2
  Cross Product : vrlib/Utilities/Cross Product
  Derivative : Derivative
  Direction Cosine Matrix to Quaternions : sharedtransform/Direction Cosine Matrix  to Quaternions  aMode=0  action=None  tolerance=eps(2)
  Dot Product : DotProduct  OutDataTypeStr=Inherit: Inherit via internal rule
  Matrix Multiply : Product  Multiplication=Matrix(*)
  Normalization1 : dspmathops/Normalization  NormType=2-norm  Bias=1e-10  NormOver=Each column  Dimension=1  roundingMode=Floor  overflowMode=off  accumDataTypeStr=Inherit: Same as product output  accumLastDataTypeStr=Inherit: Same as product output  outputDataTypeStr=Inherit: Same as product output  outputMin=[]  outputMax=[]  outputLastDataTypeStr=Inherit: Same as product output
  Normalization2 : dspmathops/Normalization  NormType=2-norm  Bias=1e-10  NormOver=Each column  Dimension=1  roundingMode=Floor  overflowMode=off  accumDataTypeStr=Inherit: Same as product output  accumLastDataTypeStr=Inherit: Same as product output  outputDataTypeStr=Inherit: Same as product output  outputMin=[]  outputMax=[]  outputLastDataTypeStr=Inherit: Same as product output
  Plus : Sum  Inputs=-+
  Product : Product
  Quaternion Inverse : aerolibutil/Quaternion Inverse
  Reshape : Reshape  OutputDimensionality=Customize  OutputDimensions=[3,3]
  Reshape1 : Reshape  OutputDimensionality=Column vector (2-D)
  Reshape2 : Reshape  OutputDimensionality=Column vector (2-D)
  Reshape3 : Reshape  OutputDimensionality=Column vector (2-D)
  Transpose : Math  Operator=transpose
  Vector Concatenate : Concatenate  NumInputs=3  Mode=Multidimensional array  ConcatenateDimension=2
  gets vector from Skew Matrix : MATLABFcn  MATLABFcn=vec_from_skew
  Q_sun_aero : Outport  VectorParamsAs1DForOutWhenUnconnected=off
  W_sun_aero : Outport  Port=2
  wires:
  Reshape2/1 -> Vector Concatenate/3, Cross Product/1
  Reshape3/1 -> Vector Concatenate/1, Cross Product/2
  Product/1 -> Plus/1
  Dot Product/1 -> Product/2
  Cross Product/1 -> Reshape1/1  "y"
  Normalization2/1 -> Reshape2/1  "z"
  Plus/1 -> Normalization2/1  "GS-(GS.x)x"
  Sun_ECI/1 -> Dot Product/2, Plus/2
  Direction Cosine Matrix to Quaternions/1 -> Quaternion Inverse/1
  Normalization1/1 -> Dot Product/1, Product/1, Reshape3/1  "x"
  <VxVyVz_ECI>/1 -> Normalization1/1
  Reshape1/1 -> Vector Concatenate/2
  Transpose/1 -> Derivative/1
  Matrix Multiply/1 -> gets vector from Skew Matrix/1
  Derivative/1 -> Matrix Multiply/1
  Vector Concatenate/1 -> Direction Cosine Matrix to Quaternions/1, Reshape/1
  gets vector from Skew Matrix/1 -> W_sun_aero/1
  Reshape/1 -> Transpose/1, Matrix Multiply/2
  Quaternion Inverse/1 -> Q_sun_aero/1

== system EPS_orbit_v5a/Attitude Reference/q_sun_aero_rotation_x_pi//1 ==
  Q_sun_aero : Inport
  Q_sun_sun : Inport  Port=2
  In3 : Inport  Port=3
  Quaternion Interpolation : QuatInterp
  Quaternion Normalize : sharedutil/Quaternion Normalize  aMode=aMode
  Quaternion Normalize1 : sharedutil/Quaternion Normalize  aMode=aMode
  Q_slerp : Outport  VectorParamsAs1DForOutWhenUnconnected=off
  wires:
  Quaternion Interpolation/1 -> Q_slerp/1
  Q_sun_sun/1 -> Quaternion Normalize1/1
  Q_sun_aero/1 -> Quaternion Normalize/1
  In3/1 -> Quaternion Interpolation/3
  Quaternion Normalize/1 -> Quaternion Interpolation/1
  Quaternion Normalize1/1 -> Quaternion Interpolation/2

== system EPS_orbit_v5a/Attitude Reference/q_sun_aero_rotation_x_pi//4 ==
  note: switch top position: no 'attitude error'
  note: this is a rotation of 45 degrees around X axis
      | to maximize the power generation, exposing faces
      | X and Y to the sun
  note: this is a rotation of 15 degrees around one axis
      | to simulate off-pointing for the power generation,
  Constant : Constant  Value=[1;0;0]
  Constant1 : Constant  Value=att.offset_axis
  Manual Switch : ManualSwitch  CurrentSetting=0
  Product : Product
  Product1 : Product
  Quaternion Multiplication : aerolibutil/Quaternion Multiplication
  Reshape1 : Reshape  OutputDimensionality=Column vector (2-D)
  Reshape2 : Reshape  OutputDimensionality=Column vector (2-D)
  Vector Concatenate1 : Concatenate  Mode=Multidimensional array
  Vector Concatenate2 : Concatenate  Mode=Multidimensional array
  cos 15 : Constant  Value=[cos(-att.offset_angle/2)]
  cos pi/2 : Constant  Value=[cos(-att.angle_roll/2)]
  sin 15 : Constant  Value=sin(-att.offset_angle/2)
  sin pi/4 : Constant  Value=sin(-att.angle_roll/2)
  Q_rot : Outport  VectorParamsAs1DForOutWhenUnconnected=off
  wires:
  cos pi/2/1 -> Vector Concatenate1/1
  Manual Switch/1 -> Q_rot/1
  sin pi/4/1 -> Product/2
  Product/1 -> Reshape1/1
  Reshape1/1 -> Vector Concatenate1/2
  Constant/1 -> Product/1  "x"
  Vector Concatenate1/1 -> Quaternion Multiplication/1, Manual Switch/1
  Product1/1 -> Reshape2/1
  cos 15/1 -> Vector Concatenate2/1
  Reshape2/1 -> Vector Concatenate2/2
  Constant1/1 -> Product1/1  "y"
  sin 15/1 -> Product1/2
  Vector Concatenate2/1 -> Quaternion Multiplication/2
  Quaternion Multiplication/1 -> Manual Switch/2

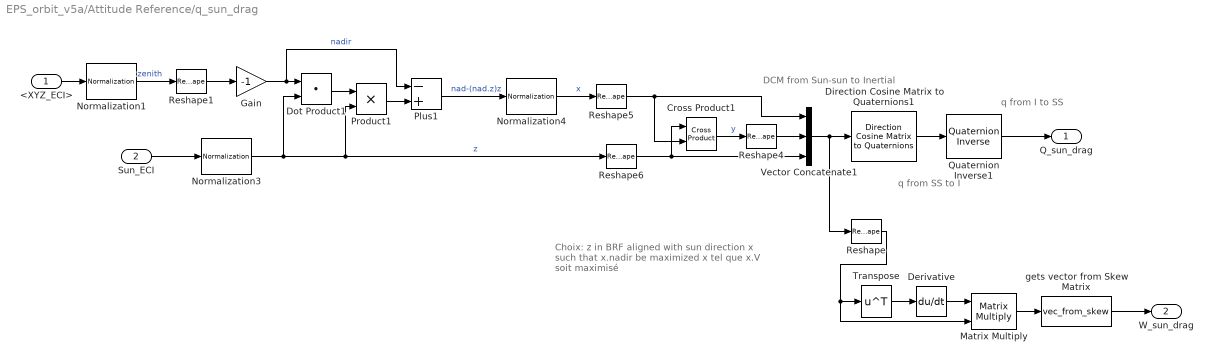
== system EPS_orbit_v5a/Attitude Reference/q_sun_drag ==
  note: Choix:
      | z in BRF aligned with sun direction
      | x such that x.nadir be maximized
      | x tel que x.V soit maximisé
  note: DCM from Sun-sun to Inertial
  note: q from I to SS
  note: q from SS to I
  <XYZ_ECI> : Inport
  Sun_ECI : Inport  Port=2
  Cross Product1 : vrlib/Utilities/Cross Product
  Derivative : Derivative
  Direction Cosine Matrix to Quaternions1 : sharedtransform/Direction Cosine Matrix  to Quaternions  aMode=0  action=None  tolerance=eps(2)
  Dot Product1 : DotProduct  OutDataTypeStr=Inherit: Inherit via internal rule
  Gain : Gain  Gain=-1
  Matrix Multiply : Product  Multiplication=Matrix(*)
  Normalization1 : dspmathops/Normalization  NormType=2-norm  Bias=1e-10  NormOver=Each column  Dimension=1  roundingMode=Floor  overflowMode=off  accumDataTypeStr=Inherit: Same as product output  accumLastDataTypeStr=Inherit: Same as product output  outputDataTypeStr=Inherit: Same as product output  outputMin=[]  outputMax=[]  outputLastDataTypeStr=Inherit: Same as product output
  Normalization3 : dspmathops/Normalization  NormType=2-norm  Bias=1e-10  NormOver=Each column  Dimension=1  roundingMode=Floor  overflowMode=off  accumDataTypeStr=Inherit: Same as product output  accumLastDataTypeStr=Inherit: Same as product output  outputDataTypeStr=Inherit: Same as product output  outputMin=[]  outputMax=[]  outputLastDataTypeStr=Inherit: Same as product output
  Normalization4 : dspmathops/Normalization  NormType=2-norm  Bias=1e-10  NormOver=Each column  Dimension=1  roundingMode=Floor  overflowMode=off  accumDataTypeStr=Inherit: Same as product output  accumLastDataTypeStr=Inherit: Same as product output  outputDataTypeStr=Inherit: Same as product output  outputMin=[]  outputMax=[]  outputLastDataTypeStr=Inherit: Same as product output
  Plus1 : Sum  Inputs=-+
  Product1 : Product
  Quaternion Inverse1 : aerolibutil/Quaternion Inverse
  Reshape : Reshape  OutputDimensionality=Customize  OutputDimensions=[3,3]
  Reshape{1,4..6} (4 alike) : Reshape  OutputDimensionality=Column vector (2-D)
  Transpose : Math  Operator=transpose
  Vector Concatenate1 : Concatenate  NumInputs=3  Mode=Multidimensional array  ConcatenateDimension=2
  gets vector from Skew Matrix : MATLABFcn  MATLABFcn=vec_from_skew
  Q_sun_drag : Outport  VectorParamsAs1DForOutWhenUnconnected=off
  W_sun_drag : Outport  Port=2
  wires:
  Direction Cosine Matrix to Quaternions1/1 -> Quaternion Inverse1/1
  Reshape4/1 -> Vector Concatenate1/2
  Dot Product1/1 -> Product1/1
  Sun_ECI/1 -> Normalization3/1
  Quaternion Inverse1/1 -> Q_sun_drag/1
  Reshape1/1 -> Gain/1
  Plus1/1 -> Normalization4/1  "nad-(nad.z)z"
  Reshape6/1 -> Cross Product1/1, Vector Concatenate1/3
  Normalization3/1 -> Dot Product1/2, Product1/2, Reshape6/1  "z"
  Reshape5/1 -> Cross Product1/2, Vector Concatenate1/1
  Cross Product1/1 -> Reshape4/1  "y"
  Normalization4/1 -> Reshape5/1  "x"
  Product1/1 -> Plus1/2
  Reshape/1 -> Matrix Multiply/2, Transpose/1
  Derivative/1 -> Matrix Multiply/1
  Transpose/1 -> Derivative/1
  Matrix Multiply/1 -> gets vector from Skew Matrix/1
  gets vector from Skew Matrix/1 -> W_sun_drag/1
  Vector Concatenate1/1 -> Direction Cosine Matrix to Quaternions1/1, Reshape/1
  <XYZ_ECI>/1 -> Normalization1/1
  Normalization1/1 -> Reshape1/1  "zenith"
  Gain/1 -> Dot Product1/1, Plus1/1  "nadir"

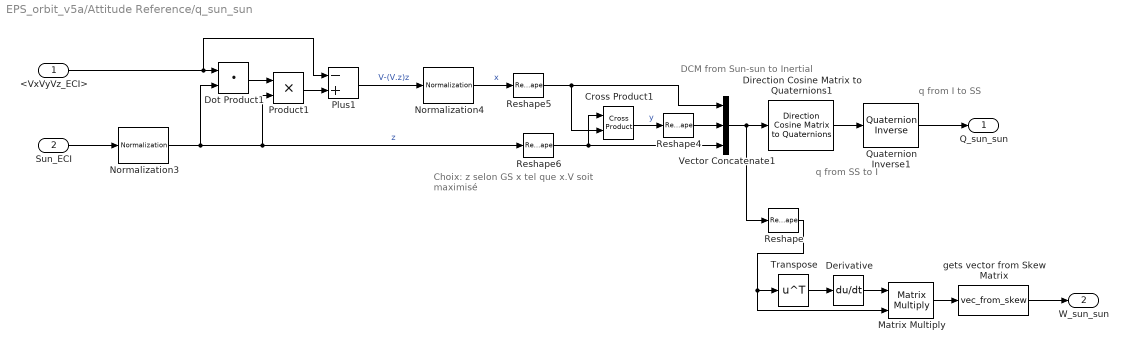
== system EPS_orbit_v5a/Attitude Reference/q_sun_sun ==
  note: Choix:
      | z selon GS
      | x tel que x.V soit maximisé
  note: DCM from Sun-sun to Inertial
  note: q from I to SS
  note: q from SS to I
  <VxVyVz_ECI> : Inport
  Sun_ECI : Inport  Port=2
  Cross Product1 : vrlib/Utilities/Cross Product
  Derivative : Derivative
  Direction Cosine Matrix to Quaternions1 : sharedtransform/Direction Cosine Matrix  to Quaternions  aMode=0  action=None  tolerance=eps(2)
  Dot Product1 : DotProduct  OutDataTypeStr=Inherit: Inherit via internal rule
  Matrix Multiply : Product  Multiplication=Matrix(*)
  Normalization3 : dspmathops/Normalization  NormType=2-norm  Bias=1e-10  NormOver=Each column  Dimension=1  roundingMode=Floor  overflowMode=off  accumDataTypeStr=Inherit: Same as product output  accumLastDataTypeStr=Inherit: Same as product output  outputDataTypeStr=Inherit: Same as product output  outputMin=[]  outputMax=[]  outputLastDataTypeStr=Inherit: Same as product output
  Normalization4 : dspmathops/Normalization  NormType=2-norm  Bias=1e-10  NormOver=Each column  Dimension=1  roundingMode=Floor  overflowMode=off  accumDataTypeStr=Inherit: Same as product output  accumLastDataTypeStr=Inherit: Same as product output  outputDataTypeStr=Inherit: Same as product output  outputMin=[]  outputMax=[]  outputLastDataTypeStr=Inherit: Same as product output
  Plus1 : Sum  Inputs=-+
  Product1 : Product
  Quaternion Inverse1 : aerolibutil/Quaternion Inverse
  Reshape : Reshape  OutputDimensionality=Customize  OutputDimensions=[3,3]
  Reshape4 : Reshape  OutputDimensionality=Column vector (2-D)
  Reshape5 : Reshape  OutputDimensionality=Column vector (2-D)
  Reshape6 : Reshape  OutputDimensionality=Column vector (2-D)
  Transpose : Math  Operator=transpose
  Vector Concatenate1 : Concatenate  NumInputs=3  Mode=Multidimensional array  ConcatenateDimension=2
  gets vector from Skew Matrix : MATLABFcn  MATLABFcn=vec_from_skew
  Q_sun_sun : Outport  VectorParamsAs1DForOutWhenUnconnected=off
  W_sun_sun : Outport  Port=2
  wires:
  Direction Cosine Matrix to Quaternions1/1 -> Quaternion Inverse1/1
  Reshape4/1 -> Vector Concatenate1/2
  Dot Product1/1 -> Product1/1
  Sun_ECI/1 -> Normalization3/1
  Quaternion Inverse1/1 -> Q_sun_sun/1
  <VxVyVz_ECI>/1 -> Dot Product1/1, Plus1/1
  Plus1/1 -> Normalization4/1  "V-(V.z)z"
  Reshape6/1 -> Cross Product1/1, Vector Concatenate1/3
  Normalization3/1 -> Dot Product1/2, Product1/2, Reshape6/1  "z"
  Reshape5/1 -> Cross Product1/2, Vector Concatenate1/1
  Cross Product1/1 -> Reshape4/1  "y"
  Normalization4/1 -> Reshape5/1  "x"
  Product1/1 -> Plus1/2
  Reshape/1 -> Matrix Multiply/2, Transpose/1
  Derivative/1 -> Matrix Multiply/1
  Transpose/1 -> Derivative/1
  Matrix Multiply/1 -> gets vector from Skew Matrix/1
  gets vector from Skew Matrix/1 -> W_sun_sun/1
  Vector Concatenate1/1 -> Direction Cosine Matrix to Quaternions1/1, Reshape/1
